simulink model "dominanciaDiagrama3"  (R2018a)
settings: Solver=VariableStepAuto  StartTime=0.0  StopTime=10  RelTol=1e-4  EnableMultiTasking=on
settings Model: Creator=fabrizio  LastModifiedBy=asm
settings DataIOCC: Refine=11
settings OptimizationCC: LifeSpan=inf
settings DebuggingCC: SFUnexpectedBacktrackingDiag=warning  SFNoUnconditionalDefaultTransitionDiag=warning  SFExecutionAtInitializationDiag=none
settings CodeAppCC: StateflowObjectComments=on
settings GRTTargetCC: TargetLangStandard=C89/C90 (ANSI)  GeneratePreprocessorConditionals=Disable all
settings ConfigComp: CovMetricSettings=dw  CovHtmlReporting=on  CovSaveCumulativeToWorkspaceVar=on  CovSaveSingleToWorkspaceVar=on  CovExternalEMLEnable=off

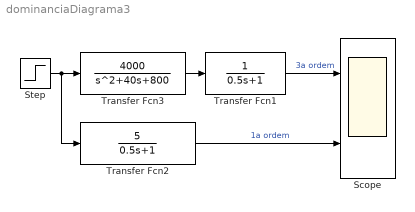
== system dominanciaDiagrama3 ==
  Scope : Scope  NumInputPorts=2
  Step : Step  After=2  SampleTime=0
  Transfer Fcn1 : TransferFcn  Denominator=[0.5 1]
  Transfer Fcn2 : TransferFcn  Numerator=[5]  Denominator=[0.5 1]
  Transfer Fcn3 : TransferFcn  Numerator=[4000]  Denominator=[1 40 800]
  wires:
  Step/1 -> Transfer Fcn2/1, Transfer Fcn3/1
  Transfer Fcn3/1 -> Transfer Fcn1/1
  Transfer Fcn1/1 -> Scope/1  "3a ordem"
  Transfer Fcn2/1 -> Scope/2  "1a ordem"
